simulink model "humidifier_humModel"  (Simulink 10.0)
settings: Solver=FixedStepAuto  StartTime=0.0  StopTime=3600  FixedStep=fixedStep  MaxStep=0.2  RelTol=1e-3
values from neighbouring files (symbols this model uses):
  massOfVapor = -30    [humidifier1Init.m]
undefined symbols (not defined in the file or in its folder): fixedStep, initMW, roomSize, startHumidifier, timeLengthHumidifier
settings Model: Creator=lixuansong  LastModifiedBy=lixuansong
settings DataIOCC: SaveFormat=Dataset  ReturnWorkspaceOutputs=on
settings OptimizationCC: LifeSpan=auto
settings DebuggingCC: UnderspecifiedInitializationDetection=Simplified  MergeDetectMultiDrivingBlocksExec=error  SFUnexpectedBacktrackingDiag=error  SFNoUnconditionalDefaultTransitionDiag=error  SFExecutionAtInitializationDiag=warning  ArithmeticOperatorsInVariantConditions=error
settings HardwareCC: ProdBitPerPointer=64  ProdBitPerSizeT=64  ProdBitPerPtrDiffT=64  ProdLargestAtomicFloat=Float  ProdIntDivRoundTo=Zero  ProdEndianess=LittleEndian  ProdWordSize=64  ProdHWDeviceType=Intel->x86-64 (Windows64)
settings ModelReferenceCC: PropagateSignalLabelsOutOfModel=on
settings SFSimCC: SimUseLocalCustomCode=on  CustomCodeUndefinedFunction=FilterOut
settings RTWCC: RTWUseLocalCustomCode=on
settings CodeAppCC: StateflowObjectComments=off
settings GRTTargetCC: TargetLangStandard=C99 (ISO)  CombineOutputUpdateFcns=on  GRTInterface=off
settings ConfigComp: CovMetricSettings=dwe  CovHtmlReporting=off  CovSaveCumulativeToWorkspaceVar=off  CovSaveSingleToWorkspaceVar=off

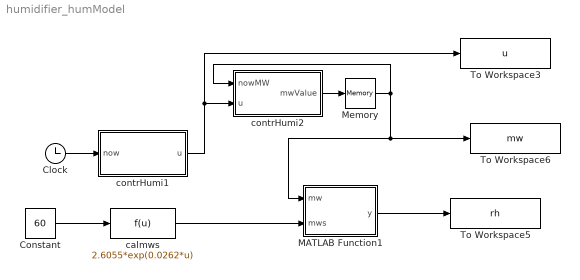
== system humidifier_humModel ==
  Clock : Clock
  Constant : Constant  Value=60
  MATLAB Function1 : MATLAB Function  TreatAsAtomicUnit=on
  Memory : Memory  InitialCondition=initMW
  To Workspace3 : ToWorkspace  VariableName=u  SampleTime=-1
  To Workspace5 : ToWorkspace  VariableName=rh  SampleTime=-1
  To Workspace6 : ToWorkspace  VariableName=mw  SampleTime=-1
  calmws : Fcn  Expr=2.6055*exp(0.0262*u)
  contrHumi1 : MATLAB Function  TreatAsAtomicUnit=on
  contrHumi2 : MATLAB Function  TreatAsAtomicUnit=on
  wires:
  Clock/1 -> contrHumi1/1(now)
  calmws/1 -> MATLAB Function1/2(mws)
  MATLAB Function1/1(y) -> To Workspace5/1
  Memory/1 -> MATLAB Function1/1(mw), To Workspace6/1, contrHumi2/1(nowMW)
  Constant/1 -> calmws/1
  contrHumi2/1(mwValue) -> Memory/1
  contrHumi1/1(u) -> To Workspace3/1, contrHumi2/2(u)

== matlab function MATLAB Function1 ==
  data: mw input double; y output double; mws input double
function y = calRH(mw,mws)

y = mw/mws;

== matlab function contrHumi1 ==
  data: u output double; now input double; startHumidifier parameter double; timeLengthHumidifier parameter double
function u = onOffHumidifier(now,startHumidifier, timeLengthHumidifier)

if (now>=startHumidifier && now<startHumidifier+timeLengthHumidifier) 
u=1;
else
    u=0;
end

== matlab function contrHumi2 ==
  data: mwValue output double; roomSize parameter double; massOfVapor parameter double; nowMW input double; u input double; fixedStep parameter double
function mwValue = controlMW(roomSize, massOfVapor, nowMW, u,fixedStep)

m=massOfVapor/roomSize/3600*fixedStep;

if u==1
    mwValue=nowMW+m;
else
    mwValue=nowMW;
end
